simulink model "pythicsmodel_freefall"  (R2023b)
settings: Solver=VariableStepAuto  StartTime=0.0  StopTime=10.0  RelTol=1e-3
settings Model: Creator=kouic  LastModifiedBy=kouic

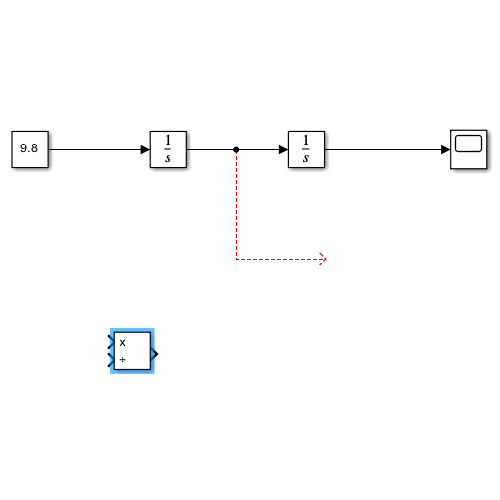
[thumbnail: Simulink's stored preview of the top-level diagram]
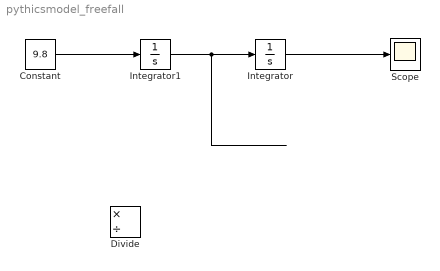
== system pythicsmodel_freefall ==
  Constant : Constant  Value=9.8
  Divide : Product  Inputs=*/
  Integrator : Integrator
  Integrator1 : Integrator
  Scope : Scope
  wires:
  Constant/1 -> Integrator1/1
  Integrator1/1 -> Integrator/1
  Integrator/1 -> Scope/1
